simulink model "motordc"  (R2013a)
settings: Solver=ode45  StartTime=0.0  StopTime=.6  RelTol=1e-3
libraries: powerlib x15, simulink x11, powerlib_extras x2
settings Model: Creator=Martial NGAHA  LastModifiedBy=leGaly

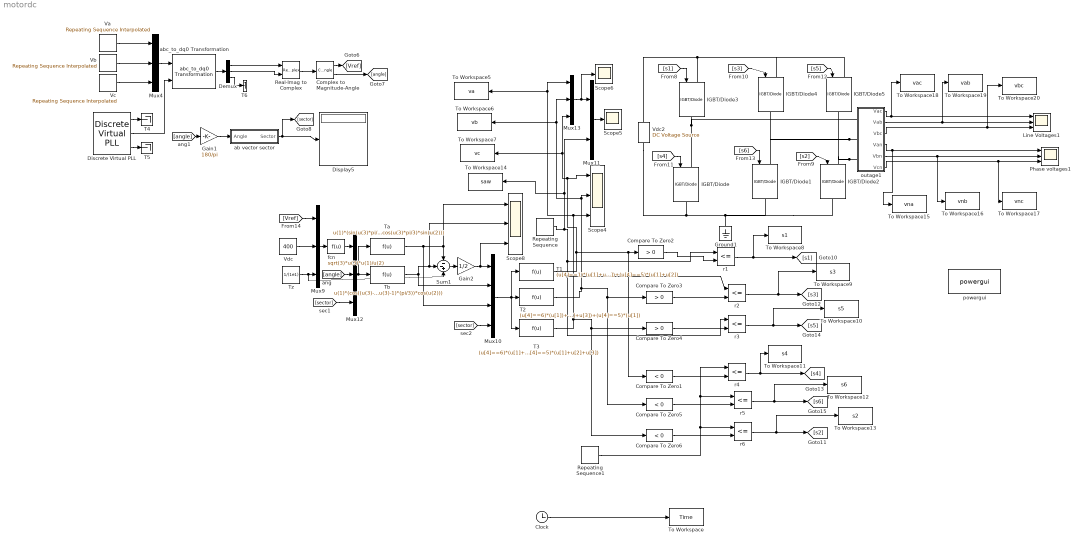
== system motordc ==
  Clock : Clock
  Compare To Zero1 : simulink/Logic and Bit Operations/Compare To Zero  relop=<  OutDataTypeStr=boolean  ZeroCross=off
  Compare To Zero2 : simulink/Logic and Bit Operations/Compare To Zero  relop=>  OutDataTypeStr=boolean  ZeroCross=off
  Compare To Zero3 : simulink/Logic and Bit Operations/Compare To Zero  relop=>  OutDataTypeStr=boolean  ZeroCross=off
  Compare To Zero4 : simulink/Logic and Bit Operations/Compare To Zero  relop=>  OutDataTypeStr=boolean  ZeroCross=off
  Compare To Zero5 : simulink/Logic and Bit Operations/Compare To Zero  relop=<  OutDataTypeStr=boolean  ZeroCross=off
  Compare To Zero6 : simulink/Logic and Bit Operations/Compare To Zero  relop=<  OutDataTypeStr=boolean  ZeroCross=off
  Complex to Magnitude-Angle : ComplexToMagnitudeAngle
  Demux : Demux  Outputs=3
  Discrete Virtual PLL : powerlib_extras/Discrete  Control Blocks/Discrete Virtual PLL  Freq=50  Phase=0  Ts=50e-6
  Display5 : Display
      settings: Decimation=6
  Gain1 : Gain  Gain=180/pi
  Gain2 : Gain  Gain=1/2
  Ground1 : powerlib/Elements/Ground  LConnTagsString=a
  IGBT/Diode{,1..5} (6 alike) : powerlib/Power Electronics/IGBT//Diode  Ron=1e-3  Rs=1e5  Cs=inf  Measurements=off
  Line Voltages1 : Scope  NumInputPorts=3
      settings: YMin=-200~-200~-200  YMax=200~200~200  SaveName=Line_voltages1  MaxDataPoints=5000000  SampleInput=on  SampleTime=2e-6
  Mux10 : Mux
  Mux11 : Mux  Inputs=2
  Mux{4,9,12..13} (4 alike) : Mux  Inputs=3
  Phase voltages1 : Scope  NumInputPorts=3
      settings: YMin=-150~-150~-150  YMax=150~150~150  SaveName=Neutral_voltages1  MaxDataPoints=5000000  SampleInput=on  SampleTime=2e-6
  Real-Imag to Complex : RealImagToComplex
  Repeating Sequence : simulink/Sources/Repeating Sequence  rep_seq_t=[0 2e-5]  rep_seq_y=[0.00001 1.5]
  Repeating Sequence1 : simulink/Sources/Repeating Sequence  rep_seq_t=[0 2e-5]  rep_seq_y=[0.00001 1.5]
  Scope4 : Scope  NumInputPorts=3
      settings: YMin=-4.06576e-020~-4.06576e-020~-4.06576e-020  YMax=0.001~0.001~0.001  SaveName=ScopeData4
  Scope5 : Scope
      settings: ShowLegends=on  YMin=0  YMax=0.001  SaveName=ScopeData5
  Scope6 : Scope
      settings: YMin=-4.06576e-020  YMax=0.001  SaveName=ScopeData6
  Scope8 : Scope  NumInputPorts=3
      settings: YMin=-5e-005~6.77626e-020~0  YMax=0.0009~0.0009~7e-005  SaveName=ScopeData7
  Sum1 : Sum  Inputs=--+
  T1 : Fcn  Expr=(u[4]==1)*(u[1]+u[2]+u[3])+(u[4]==6)*(u[1]+u[2]+u[3])+(u[4]==2)*(u[1]+u[3])+(u[4]==3)*(u[1])+(u[4]==4)*(u[1])+(u[4]==5)*(u[1]+u[2])
  T2 : Fcn  Expr=(u[4]==6)*(u[1])+(u[4]==1)*(u[1]+u[2])+(u[4]==2)*(u[1]+u[2]+u[3])+(u[4]==3)*(u[1]+u[2]+u[3])+(u[4]==4)*(u[1]+u[3])+(u[4]==5)*(u[1])
  T3 : Fcn  Expr=(u[4]==6)*(u[1]+u[3])+(u[4]==1)*(u[1])+(u[4]==2)*(u[1])+(u[4]==3)*(u[1]+u[2])+(u[4]==4)*(u[1]+u[2]+u[3])+(u[4]==5)*(u[1]+u[2]+u[3])
  T4 : Terminator
  T5 : Terminator
  T6 : Terminator
  Ta : Fcn  Expr=u(1)*(sin(u(3)*pi/3)*cos(u(2))-cos(u(3)*pi/3)*sin(u(2)))
  Tb : Fcn  Expr=u(1)*(cos((u(3)-1)*(pi/3))*sin(u(2))-sin((u(3)-1)*(pi/3))*cos(u(2)))
  To Workspace : ToWorkspace  VariableName=Time  SampleTime=-1  SaveFormat=Structure With Time
  To Workspace10 : ToWorkspace  VariableName=s5  SampleTime=-1  SaveFormat=Structure With Time
  To Workspace11 : ToWorkspace  VariableName=s4  SampleTime=-1  SaveFormat=Structure With Time
  To Workspace12 : ToWorkspace  VariableName=s6  SampleTime=-1  SaveFormat=Structure With Time
  To Workspace13 : ToWorkspace  VariableName=s2  SampleTime=-1  SaveFormat=Structure With Time
  To Workspace14 : ToWorkspace  VariableName=saw  SampleTime=-1  SaveFormat=Structure With Time
  To Workspace15 : ToWorkspace  VariableName=vna  SampleTime=-1  SaveFormat=Structure With Time
  To Workspace16 : ToWorkspace  VariableName=vnb  SampleTime=-1  SaveFormat=Structure With Time
  To Workspace17 : ToWorkspace  VariableName=vnc  SampleTime=-1  SaveFormat=Structure With Time
  To Workspace18 : ToWorkspace  VariableName=vac  SampleTime=-1  SaveFormat=Structure With Time
  To Workspace19 : ToWorkspace  VariableName=vab  SampleTime=-1  SaveFormat=Structure With Time
  To Workspace20 : ToWorkspace  VariableName=vbc  SampleTime=-1  SaveFormat=Structure With Time
  To Workspace5 : ToWorkspace  VariableName=va  SampleTime=-1  SaveFormat=Structure With Time
  To Workspace6 : ToWorkspace  VariableName=vb  SampleTime=-1  SaveFormat=Structure With Time
  To Workspace7 : ToWorkspace  VariableName=vc  SampleTime=-1  SaveFormat=Structure With Time
  To Workspace8 : ToWorkspace  VariableName=s1  SampleTime=-1  SaveFormat=Structure With Time
  To Workspace9 : ToWorkspace  VariableName=s3  SampleTime=-1  SaveFormat=Structure With Time
  Tz : Constant  Value=1/(1e1)
  "Va " : simulink/Sources/Repeating Sequence Interpolated  OutValues=[250 250 -250 -250 250 250 -250 -250].'  TimeValues=[0 0.2 0.3 0.5 0.6 0.8 0.9 1.1].'  LookUpMeth=Interpolation-Use End Values  tsamp=0.01  OutMin=[]  OutMax=[]  OutDataTypeStr=double  OutputDataTypeScalingMode=double  OutDataType=fixdt(0,8)  OutScaling=2^-10
  Vb : simulink/Sources/Repeating Sequence Interpolated  OutValues=[-250 -250 250 250 -250 -250 250 250].'  TimeValues=[0 0.1 0.2 0.4 0.5 0.7 0.8 1 ].'  LookUpMeth=Interpolation-Use End Values  tsamp=0.01  OutMin=[]  OutMax=[]  OutDataTypeStr=double  OutputDataTypeScalingMode=double  OutDataType=fixdt(0,8)  OutScaling=2^-10
  Vc : simulink/Sources/Repeating Sequence Interpolated  OutValues=[250 -250 -250 250 250 -250 -250 250].'  TimeValues=[0 0.1 0.3 0.4 0.6 0.7 0.9 1].'  LookUpMeth=Interpolation-Use End Values  tsamp=0.01  OutMin=[]  OutMax=[]  OutDataTypeStr=double  OutputDataTypeScalingMode=double  OutDataType=fixdt(0,8)  OutScaling=2^-10
  Vdc : Constant  Value=400
  Vdc2 : powerlib/Electrical Sources/DC Voltage Source  Amplitude=400  Measurements=None
  ab vector sector : Subsystem  AncestorBlock=AC2DriveInternalModels/SVM generator/ab vector sector
  abc_to_dq0 Transformation : powerlib_extras/Measurements/abc_to_dq0 Transformation
  fcn : Fcn  Expr=sqrt(3)*u(3)*u(1)/u(2)
  outage1 : Subsystem
  powergui : powerlib/powergui  Priority=1  SimulationMode=Discrete  SolverType=Tustin  SampleTime=1e-6  frequency=60  SPID=off  DisableSnubberDevices=off  DisableRonSwitches=off  DisableVfSwitches=off  SwTol=0  Interpol=off  DisplayEquations=off  frequencyindice=0  Pbase=100e6  ErrMax=1e-4  Iterations=50  UnitsV=kV  UnitsW=MW  FunctionMessages=off  echomessages=off  HookPort=off  EnableUseOfTLC=off  x0status=blocks  RestoreLinks=warning  ResistiveCurrentMeasurement=off  Frange=[0:2:500]  Ylog=off  Xlog=on  ShowGrid=off  save=off  variable=ZData  structure=Neutral_voltages  ZoomFFT=off  StartTime=0  cycles=1  DisplayStyle=3  fundamental=50  FreqAxis=off  MaxFrequency=200  frequencyindicesteady=1  RmsSteady=1  display=off  Ts=0  methode=off
  r{1..6} (6 alike) : RelationalOperator  Operator=<=  OutDataTypeStr=boolean
  wires:
  Discrete Virtual PLL/2 -> abc_to_dq0 Transformation/2
  abc_to_dq0 Transformation/1 -> Demux/1
  Demux/1 -> Real-Imag to Complex/1
  Demux/2 -> Real-Imag to Complex/2
  Real-Imag to Complex/1 -> Complex to Magnitude-Angle/1
  Discrete Virtual PLL/3 -> T5/1
  Discrete Virtual PLL/1 -> T4/1
  "Va "/1 -> Mux4/1
  Gain1/1 -> ab vector sector/1(Angle)
  Complex to Magnitude-Angle/2 -> [angle]
  ab vector sector/1(Sector) -> Display5/1, [sector]
  Mux4/1 -> abc_to_dq0 Transformation/1
  Demux/3 -> T6/1
  Complex to Magnitude-Angle/1 -> [Vref]
  [angle] -> Gain1/1
  Vb/1 -> Mux4/2
  Vc/1 -> Mux4/3
  Ta/1 -> Mux10/3, Sum1/1, Scope8/1
  Tb/1 -> Sum1/2, Scope8/2, Mux10/2
  Vdc/1 -> Mux9/2
  Tz/1 -> Mux9/3, Sum1/3
  Mux9/1 -> fcn/1
  fcn/1 -> Mux12/1
  Mux12/1 -> Ta/1, Tb/1
  Sum1/1 -> Gain2/1
  Gain2/1 -> Mux10/1, Scope8/3
  Mux10/1 -> T2/1, T1/1, T3/1
  r1/1 -> To Workspace8/1, [s1]
  r2/1 -> To Workspace9/1, [s3]
  r3/1 -> To Workspace10/1, [s5]
  Mux13/1 -> Mux11/1, Scope6/1
  Repeating Sequence/1 -> r1/1, r2/1, r3/1, To Workspace14/1, Mux11/2
  T1/1 -> Compare To Zero1/1, Compare To Zero2/1, To Workspace7/1, Mux13/3, Scope4/1
  T2/1 -> Compare To Zero5/1, Compare To Zero3/1, Scope4/2, Mux13/2, To Workspace6/1
  T3/1 -> Compare To Zero6/1, Compare To Zero4/1, Scope4/3, To Workspace5/1, Mux13/1
  Mux11/1 -> Scope5/1
  [s1] -> IGBT/Diode3/1
  [s3] -> IGBT/Diode4/1
  [s6] -> IGBT/Diode1/1
  [s5] -> IGBT/Diode5/1
  [s2] -> IGBT/Diode2/1
  outage1/4(Van) -> Phase voltages1/1, To Workspace15/1
  outage1/5(Vbn) -> To Workspace16/1, Phase voltages1/2
  outage1/6(Vcn) -> To Workspace17/1, Phase voltages1/3
  outage1/1(Vac) -> To Workspace18/1, Line Voltages1/1
  outage1/2(Vab) -> To Workspace19/1, Line Voltages1/2
  outage1/3(Vbc) -> To Workspace20/1, Line Voltages1/3
  [s4] -> IGBT/Diode/1
  [Vref] -> Mux9/1
  [angle] -> Mux12/2
  [sector] -> Mux12/3
  [sector] -> Mux10/4
  Clock/1 -> To Workspace/1
  r6/1 -> To Workspace13/1, [s2]
  r5/1 -> To Workspace12/1, [s6]
  r4/1 -> To Workspace11/1, [s4]
  Repeating Sequence1/1 -> r4/1, r5/1, r6/1
  Compare To Zero1/1 -> r4/2
  Compare To Zero5/1 -> r5/2
  Compare To Zero6/1 -> r6/2
  Compare To Zero2/1 -> r1/2
  Compare To Zero3/1 -> r2/2
  Compare To Zero4/1 -> r3/2
  connections:
  Vdc2/RConn1 -- IGBT/Diode3/LConn1 -- IGBT/Diode5/LConn1 -- IGBT/Diode4/LConn1
  IGBT/Diode/LConn1 -- outage1/LConn1 -- IGBT/Diode3/RConn1
  outage1/LConn3 -- IGBT/Diode5/RConn1 -- IGBT/Diode2/LConn1
  IGBT/Diode2/RConn1 -- IGBT/Diode1/RConn1 -- Ground1/LConn1 -- IGBT/Diode/RConn1 -- Vdc2/LConn1
  outage1/LConn2 -- IGBT/Diode4/RConn1 -- IGBT/Diode1/LConn1

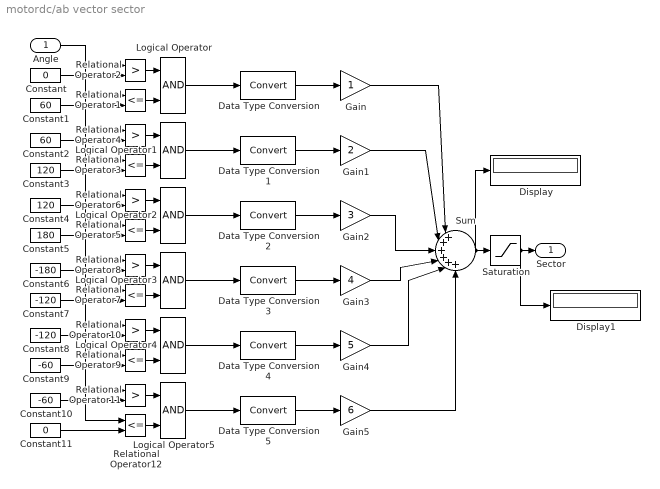
== system motordc/ab vector sector ==
  Angle : Inport
  Constant : Constant  Value=0
  Constant1 : Constant  Value=60
  Constant10 : Constant  Value=-60
  Constant11 : Constant  Value=0
  Constant2 : Constant  Value=60
  Constant3 : Constant  Value=120
  Constant4 : Constant  Value=120
  Constant5 : Constant  Value=180
  Constant6 : Constant  Value=-180
  Constant7 : Constant  Value=-120
  Constant8 : Constant  Value=-120
  Constant9 : Constant  Value=-60
  Data Type Conversion{,1..5} (6 alike) : DataTypeConversion  SaturateOnIntegerOverflow=on  RndMeth=Zero
  Display : Display
  Display1 : Display
  Gain : Gain  SaturateOnIntegerOverflow=on  OutDataTypeStr=Inherit: Same as input  ParamDataTypeStr=Inherit: Same as input
  Gain1 : Gain  Gain=2  SaturateOnIntegerOverflow=on  OutDataTypeStr=Inherit: Same as input  ParamDataTypeStr=Inherit: Same as input
  Gain2 : Gain  Gain=3  SaturateOnIntegerOverflow=on  OutDataTypeStr=Inherit: Same as input  ParamDataTypeStr=Inherit: Same as input
  Gain3 : Gain  Gain=4  SaturateOnIntegerOverflow=on  OutDataTypeStr=Inherit: Same as input  ParamDataTypeStr=Inherit: Same as input
  Gain4 : Gain  Gain=5  SaturateOnIntegerOverflow=on  OutDataTypeStr=Inherit: Same as input  ParamDataTypeStr=Inherit: Same as input
  Gain5 : Gain  Gain=6  SaturateOnIntegerOverflow=on  OutDataTypeStr=Inherit: Same as input  ParamDataTypeStr=Inherit: Same as input
  Logical Operator{,1..5} (6 alike) : Logic
  Relational Operator{1,3,5,7,9,12} (6 alike) : RelationalOperator  Operator=<=  InputSameDT=on
  Relational Operator{2,4,6,8,10..11} (6 alike) : RelationalOperator  Operator=>  InputSameDT=on
  Saturation : Saturate  UpperLimit=6  LowerLimit=1
  Sum : Sum  Inputs=|++++++  SaturateOnIntegerOverflow=on  InputSameDT=on  OutDataTypeStr=Inherit: Same as first input
  Sector : Outport
  wires:
  Data Type Conversion5/1 -> Gain5/1
  Data Type Conversion4/1 -> Gain4/1
  Data Type Conversion3/1 -> Gain3/1
  Data Type Conversion2/1 -> Gain2/1
  Data Type Conversion1/1 -> Gain1/1
  Data Type Conversion/1 -> Gain/1
  Relational Operator2/1 -> Logical Operator/1
  Relational Operator1/1 -> Logical Operator/2
  Logical Operator/1 -> Data Type Conversion/1
  Angle/1 -> Relational Operator2/1, Relational Operator1/1, Relational Operator4/1, Relational Operator3/1, Relational Operator6/1, Relational Operator5/1, Relational Operator8/1, Relational Operator7/1, Relational Operator10/1, Relational Operator9/1, Relational Operator11/1, Relational Operator12/1
  Constant/1 -> Relational Operator2/2
  Constant1/1 -> Relational Operator1/2
  Relational Operator4/1 -> Logical Operator1/1
  Relational Operator3/1 -> Logical Operator1/2
  Logical Operator1/1 -> Data Type Conversion1/1
  Constant2/1 -> Relational Operator4/2
  Constant3/1 -> Relational Operator3/2
  Relational Operator6/1 -> Logical Operator2/1
  Relational Operator5/1 -> Logical Operator2/2
  Logical Operator2/1 -> Data Type Conversion2/1
  Constant4/1 -> Relational Operator6/2
  Constant5/1 -> Relational Operator5/2
  Relational Operator8/1 -> Logical Operator3/1
  Relational Operator7/1 -> Logical Operator3/2
  Logical Operator3/1 -> Data Type Conversion3/1
  Constant6/1 -> Relational Operator8/2
  Constant7/1 -> Relational Operator7/2
  Relational Operator10/1 -> Logical Operator4/1
  Relational Operator9/1 -> Logical Operator4/2
  Logical Operator4/1 -> Data Type Conversion4/1
  Constant8/1 -> Relational Operator10/2
  Constant9/1 -> Relational Operator9/2
  Relational Operator11/1 -> Logical Operator5/1
  Relational Operator12/1 -> Logical Operator5/2
  Logical Operator5/1 -> Data Type Conversion5/1
  Constant10/1 -> Relational Operator11/2
  Constant11/1 -> Relational Operator12/2
  Gain/1 -> Sum/1
  Gain1/1 -> Sum/2
  Gain2/1 -> Sum/3
  Gain3/1 -> Sum/4
  Gain4/1 -> Sum/5
  Gain5/1 -> Sum/6
  Sum/1 -> Saturation/1, Display/1
  Saturation/1 -> Sector/1, Display1/1

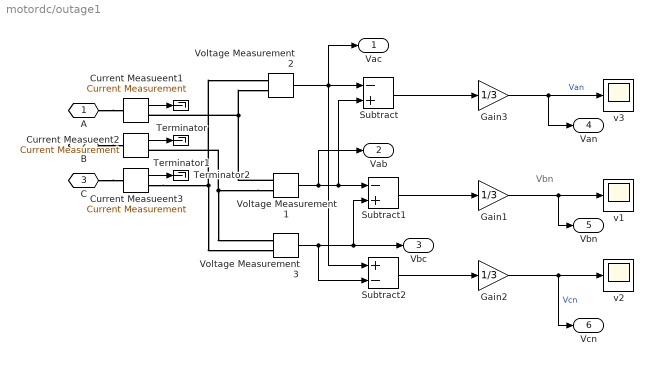
== system motordc/outage1 ==
  note: Vbn
  Current Measueent1 : powerlib/Measurements/Current Measurement  PhasorSimulation=off  OutputType=Complex  PSBequivalent=0
  Current Measueent2 : powerlib/Measurements/Current Measurement  PhasorSimulation=off  OutputType=Complex  PSBequivalent=0
  Current Measueent3 : powerlib/Measurements/Current Measurement  PhasorSimulation=off  OutputType=Complex  PSBequivalent=0
  Gain1 : Gain  Gain=1/3
  Gain2 : Gain  Gain=1/3
  Gain3 : Gain  Gain=1/3
  Subtract : Sum  Inputs=-+
  Subtract1 : Sum  Inputs=-+
  Subtract2 : Sum  Inputs=+-
  Terminator : Terminator
  Terminator1 : Terminator
  Terminator2 : Terminator
  Voltage Measurement1 : powerlib/Measurements/Voltage Measurement  PhasorSimulation=off  OutputType=Complex  PSBequivalent=0
  Voltage Measurement2 : powerlib/Measurements/Voltage Measurement  PhasorSimulation=off  OutputType=Complex  PSBequivalent=0
  Voltage Measurement3 : powerlib/Measurements/Voltage Measurement  PhasorSimulation=off  OutputType=Complex  PSBequivalent=0
  v1 : Scope
      settings: SaveName=ScopeData25  MaxDataPoints=5000000
  v2 : Scope
      settings: SaveName=ScopeData26  MaxDataPoints=5000000
  v3 : Scope
      settings: YMin=-25  YMax=275  SaveName=ScopeData27  MaxDataPoints=5000000
  A : PMIOPort  Port=1  Side=Left
  B : PMIOPort  Port=2  Side=Left
  C : PMIOPort  Port=3  Side=Left
  Vac : Outport
  Vab : Outport  Port=2
  Vbc : Outport  Port=3
  Van : Outport  Port=4
  Vbn : Outport  Port=5
  Vcn : Outport  Port=6
  wires:
  Gain2/1 -> v2/1, Vcn/1  "Vcn"
  Subtract2/1 -> Gain2/1
  Gain1/1 -> v1/1, Vbn/1
  Subtract1/1 -> Gain1/1
  Voltage Measurement3/1 -> Subtract2/2, Subtract1/2, Vbc/1
  Gain3/1 -> v3/1, Van/1  "Van"
  Subtract/1 -> Gain3/1
  Voltage Measurement1/1 -> Subtract/2, Subtract1/1, Vab/1
  Voltage Measurement2/1 -> Subtract/1, Subtract2/1, Vac/1
  Current Measueent1/1 -> Terminator/1
  Current Measueent2/1 -> Terminator1/1
  Current Measueent3/1 -> Terminator2/1
  connections:
  Voltage Measurement1/LConn1 -- Current Measueent1/RConn1 -- Voltage Measurement2/LConn2
  Voltage Measurement1/LConn2 -- Current Measueent2/RConn1 -- Voltage Measurement3/LConn1
  Current Measueent3/RConn1 -- Voltage Measurement2/LConn1 -- Voltage Measurement3/LConn2
  A/RConn1 -- Current Measueent1/LConn1
  B/RConn1 -- Current Measueent2/LConn1
  C/RConn1 -- Current Measueent3/LConn1
